simulink model "simvib"  (R2016a)
settings: Solver=FixedStepDiscrete  StartTime=0.0  StopTime=inf  FixedStep=0.01  RelTol=1e-3
undefined symbols (not defined in the file or in its folder): getvib
settings Model: Creator=Edzko  LastModifiedBy=Edzko

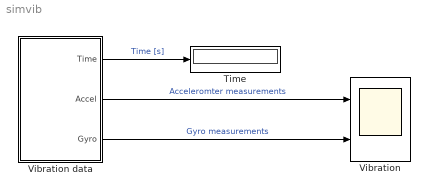
== system simvib ==
  Time : Display
      settings: Format=bank
  Vibration : Scope  NumInputPorts=2
  Vibration data : Subsystem  LoadFcn=set_param(gcb,'Maskstylestring',['popup(',acc('LIST'),'),popup(230400|115200|57600|38400|19200|14400|9600)'])  mask{comport=USB Serial Device (COM19), baud=115200}
      mask prompts: comport "Com port:"; baud "Baudrate:"
      mask init:
      | acc(comport)
      mask TypeOptions comport: USB Serial Device (COM13) | USB Serial Device (COM19) | Prolific USB-to-Serial Comm Port (COM20) | USB Serial Port (COM26) | USB Serial Port (COM27) | USB Serial Port (COM28) | USB Serial Port (COM29) | Prolific USB-to-Serial Comm Port (COM14) | IP:192.168.1.1
      mask TypeOptions baud: 230400 | 115200 | 57600 | 38400 | 19200 | 14400 | 9600
  wires:
  Vibration data/1(Time) -> Time/1  "Time [s]"
  Vibration data/2(Accel) -> Vibration/1  "Acceleromter measurements"
  Vibration data/3(Gyro) -> Vibration/2  "Gyro measurements"

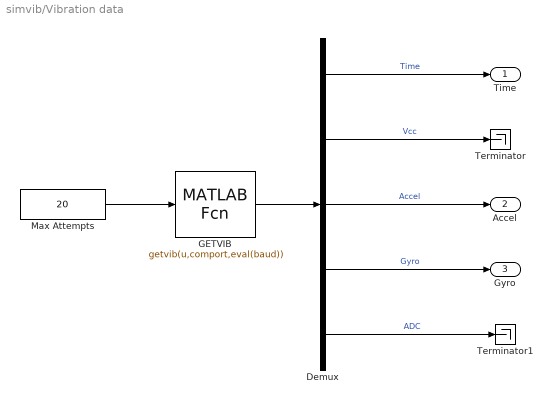
== system simvib/Vibration data ==
  Demux : Demux  Outputs=[1 1 3 3 4]
  GETVIB : MATLABFcn  MATLABFcn=getvib(u,comport,eval(baud))  OutputDimensions=12
  Max Attempts : Constant  Value=20
  Terminator : Terminator
  Terminator1 : Terminator
  Time : Outport
  Accel : Outport  Port=2
  Gyro : Outport  Port=3
  wires:
  Demux/3 -> Accel/1  "Accel"
  Demux/1 -> Time/1  "Time"
  Demux/2 -> Terminator/1  "Vcc"
  Demux/4 -> Gyro/1  "Gyro"
  GETVIB/1 -> Demux/1
  Demux/5 -> Terminator1/1  "ADC"
  Max Attempts/1 -> GETVIB/1
